simulink model "SingleTrackCANoe"  (R2021b)
settings: Solver=ode1  StartTime=0  StopTime=2  FixedStep=1.0000000000000000e-003  RelTol=1e-3
InitFcn:
  | sampleTime = str2double(get_param(bdroot, 'FixedStep'));
undefined symbols (not defined in the file or in its folder): AccPedalPos, BrakePedalPos, BrakeSwitch, DiscIntNeverNeededParam, DYNA4, EngSpd, IgnitionSwitch, InitialGear, InitialSpeed, IntendedEngTrq, LeftIndicator, MainBrakePress, MaxGear, MDL, MinGear, RefAcc, RefLane, RefLatPos, RefPath, RefPathCurv, RefSpd, RefSpdPreview, RefSpdRetrospect, RightIndicator, SteeringWheelAng, SteeringWheelTrq, UserDefinedRefValue, vm_const
libraries: UtilitiesLibrary x62, simulink x18, WheelSystemModules x14, LongitudinalControllerModules x13, LateralControllerModules x7, AnimationBusselectorModules x5, EnvironmentModules x5, BasicEngineControlModules x5, MiscellaneousControlModules x5, Animation3Modules x4, AuxiliariesModules x4, ReducedTireModules x4
(part 2 of 34)

== system SingleTrackCANoe/SimulationModel ==
  note: Update Switch Board Connections
  Enable : EnablePort  StatesWhenEnabling=reset
  Animation : Subsystem
  ComponentsOutput : Subsystem  Tag=TESIS DYNAware Interface Block  mask{NeedsUpdate=off, SignalInfo=|}
      mask SignalInfo=|
      | {
      |   "Version": "4.6",
      |   "MuxedOutputBusName": "Components",
      |   "MuxedInputBusName": "input",
      |   "MuxedInputSelected": false,
      |   "MuxedOutputSelected": true,
      |   "SignalData": [
      |     {
      |       "initialValue": "0.0",
      |       "name": "",
      |       "comment": "",
      |       "minString": "",
      |       "maxString": "",
      |       "width": 1,
      |       "dataType": 0,
      |       "signalType": 0,
      |       "createSignal": true,
      |       "outputName": "(none)",
      |       "generateSignalAccessBlock": false,
      |       "accessId": "$(parentId).$(blockName).$(outputName)"
      |     },
      |     {
      |       "initialValue": "0.0",
      |       "name": "ControlUnits",
      |       "comment": "",
      |       "minString": "",
      |       "maxString": "",
      |       "width": -1,
      |       "dataType": 0,
      |       "signalType": 1,
      |       "createSignal": false,
      |       "outputName": "ControlUnits",
      |       "generateSignalAccessBlock": false,
      |       "accessId": "$(parentId).$(blockName).$(outputName)"
      |     },
      |     {
      |       "initialValue": "0.0",
      |       "name": "Trailer",
      |       "comment": "",
      |       "minString": "",
      |       "maxString": "",
      |       "width": -1,
      |       "dataType": 0,
      |       "signalType": 1,
      |       "createSignal": false,
      |       "outputName": "Trailer",
      |       "generateSignalAccessBlock": false,
      |       "accessId": "$(parentId).$(blockName).$(outputName)"
      |     },
      |     {
      |       "initialValue": "0.0",
      |       "name": "Vehicle",
      |       "comment": "",
      |       "minString": "",
      |       "maxString": "",
      |       "width": -1,
      |       "dataType": 0,
      |       "signalType": 1,
      |       "createSignal": false,
      |       "outputName": "Vehicle",
      |       "generateSignalAccessBlock": false,
      |       "accessId": "$(parentId).$(blockName).$(outputName)"
      |     },
      |     {
      |       "initialValue": "0.0",
      |       "name": "Environment",
      |       "comment": "",
      |       "minString": "",
      |       "maxString": "",
      |       "width": -1,
      |       "dataType": 0,
      |       "signalType": 1,
      |       "createSignal": false,
      |       "outputName": "Environment",
      |       "generateSignalAccessBlock": false,
      |       "accessId": "$(parentId).$(blockName).$(outputName)"
      |     },
      |     {
      |       "initialValue": "0.0",
      |       "name": "Traffic",
      |       "comment": "",
      |       "minString": "",
      |       "maxString": "",
      |       "width": -1,
      |       "dataType": 0,
      |       "signalType": 1,
      |       "createSignal": false,
      |       "outputName": "Traffic",
      |       "generateSignalAccessBlock": false,
      |       "accessId": "$(parentId).$(blockName).$(outputName)"
      |     },
      |     {
      |       "initialValue": "0.0",
      |       "name": "VehicleControl",
      |       "comment": "",
      |       "minString": "",
      |       "maxString": "",
      |       "width": -1,
      |       "dataType": 0,
      |       "signalType": 1,
      |       "createSignal": false,
      |       "outputName": "VehicleControl",
      |       "generateSignalAccessBlock": false,
      |       "accessId": "$(parentId).$(blockName).$(outputName)"
      |     }
      |   ]
      | }
      mask prompts: NeedsUpdate "Specify, if subsystem content needs to be updated"; SignalInfo "Signal Info (json)"
      mask help: DYNA4 Interface Block Version 4.6
      mask init:
      | blockName = get_param(gcbh, 'Name');
      | parentId = DYNA4.ModelHandling.AccessID.getFromHierarchy(gcbh);
      | TD.InterfaceBlock.ModelCallbacks.GenerateContent(gcb);
      settings: AttributesFormatString=(none) = 0.0  DeleteFcn=TD.InterfaceBlock.ModelCallbacks.CloseGUI( gcbh );  NameChangeFcn=TD.InterfaceBlock.ModelCallbacks.BlockRenamedHandler(gcbh);  OpenFcn=TD.InterfaceBlock.ModelCallbacks.OpenGUI( gcbh );  CloseFcn=TD.InterfaceBlock.ModelCallbacks.CloseGUI( gcbh );
      mask Display:
      | image('InterfaceBlock.png','center');
      | port_label('input',1, 'ControlUnits');
      | port_label('input',2, 'Trailer');
      | port_label('input',3, 'Vehicle');
      | port_label('input',4, 'Environment');
      | port_label('input',5, 'Traffic');
      | port_label('input',6, 'VehicleControl');
      | port_label('output',1, 'Components');
  ControlUnits : Subsystem
  DYNA4 Logo : Subsystem
      settings: AttributesFormatString=DYNA4 Version: 9.1
      settings: PreSaveFcn=|
      | try
      |   set_param(gcb,'AttributesFormatString',['DYNA4 Version: ' dm_get_model_version(bdroot)]);
      | end
      mask Display: image('DYNA4_Model_Splash.jpg');
  Environment : Subsystem
  SwitchBoard : Subsystem  Tag=DYNA4SwitchBoard  mask{NeedsUpdate=off, SignalInfo=|}
      mask SignalInfo=|
      | {
      |   "Version": "4.6",
      |   "MuxedOutputBusName": "CTRL",
      |   "MuxedInputBusName": "Components",
      |   "MuxedInputSelected": true,
      |   "MuxedOutputSelected": true,
      |   "SignalData": [
      |     {
      |       "initialValue": "0.0",
      |       "name": "Environment.AdditionalRoadElevation.AddLatRoadSlope[-]",
      |       "comment": "",
      |       "minString": "",
      |       "maxString": "",
      |       "width": -1,
      |       "dataType": 0,
      |       "signalType": 0,
      |       "createSignal": false,
      |       "outputName": "CTRL.AdditionalRoadElevation.AddLatRoadSlope[-]",
      |       "generateSignalAccessBlock": false,
      |       "accessId": "$(outputName)"
      |     },
      |     {
      |       "initialValue": "0.0",
      |       "name": "Environment.AdditionalRoadElevation.AddLongRoadSlope[-]",
      |       "comment": "",
      |       "minString": "",
      |       "maxString": "",
      |       "width": -1,
      |       "dataType": 0,
      |       "signalType": 0,
      |       "createSignal": false,
      |       "outputName": "CTRL.AdditionalRoadElevation.AddLongRoadSlope[-]",
      |       "generateSignalAccessBlock": false,
      |       "accessId": "$(outputName)"
      |     },
      |     {
      |       "initialValue": "0.0 (auto grounded)",
      |       "name": "",
      |       "comment": "",
      |       "minString": "",
      |       "maxString": "",
      |       "width": 1,
      |       "dataType": 0,
      |       "signalType": 0,
      |       "createSignal": true,
      |       "outputName": "CTRL.AdditionalRoadElevation.ExternalAddLatRoadSlopeEnforced",
      |       "generateSignalAccessBlock": true,
      |       "accessId": "$(outputName)"
      |     },
      |     {
      |       "initialValue": "0.0 (auto grounded)",
      |       "name": "",
      |       "comment": "",
      |       "minString": "",
      |       "maxString": "",
      |       "width": 1,
      |       "dataType": 0,
      |       "signalType": 0,
      |       "createSignal": true,
      |       "outputName": "CTRL.AdditionalRoadElevation.ExternalAddLatRoadSlope[-]",
      |       "generateSignalAccessBlock": false,
      |       "accessId": "$(outputName)"
      |     },
      |     {
      |       "initialValue": "0.0 (auto grounded)",
      |       "name": "",
      |       "comment": "",
      |       "minString": "",
      |       "maxString": "",
      |       "width": 1,
      |       "dataType": 0,
      |       "signalType": 0,
      |       "createSignal": true,
      |       "outputName": "CTRL.AdditionalRoadElevation.ExternalAddLongRoadSlopeEnforced",
      |       "generateSignalAccessBlock": true,
      |       "accessId": "$(outputName)"
      |     },
      |     {
      |       "initialValue": "0.0 (auto grounded)",
      |       "name": "",
      |       "comment": "",
      |       "minString": "",
      |       "maxString": "",
      |       "width": 1,
      |       "dataType": 0,
      |       "signalType": 0,
      |       "createSignal": true,
      |       "outputName": "CTRL.AdditionalRoadElevation.ExternalAddLongRoadSlope[-]",
      |       "generateSignalAccessBlock": false,
      |       "accessId": "$(outputName)"
      |     },
      |     {
      |       "initialValue": "0.0",
      |       "name": "Environment.AdditionalRoadElevation.FrontLeftAddLatRoadSlope[-]",
      |       "comment": "",
      |       "minString": "",
      |       "maxString": "",
      |       "width": 1,
      |       "dataType": 0,
      |       "signalType": 0,
      |       "createSignal": false,
      |       "outputName": "CTRL.AdditionalRoadElevation.FrontLeftAddLatRoadSlope[-]",
      |       "generateSignalAccessBlock": false,
      |       "accessId": "$(outputName)"
      |     },
      |     {
      |       "initialValue": "0.0",
      |       "name": "Environment.AdditionalRoadElevation.FrontLeftAddLongRoadSlope[-]",
      |       "comment": "",
      |       "minString": "",
      |       "maxString": "",
      |       "width": 1,
      |       "dataType": 0,
      |       "signalType": 0,
      |       "createSignal": false,
      |       "outputName": "CTRL.AdditionalRoadElevation.FrontLeftAddLongRoadSlope[-]",
      |       "generateSignalAccessBlock": false,
      |       "accessId": "$(outputName)"
      |     },
      |     {
      |       "initialValue": "0.0",
      |       "name": "Environment.AdditionalRoadElevation.FrontLeftAddRoadElev[m]",
      |       "comment": "",
      |       "minString": "",
      |       "maxString": "",
      |       "width": -1,
      |       "dataType": 0,
      |       "signalType": 0,
      |       "createSignal": false,
      |       "outputName": "CTRL.AdditionalRoadElevation.FrontLeftAddRoadElev[m]",
      |       "generateSignalAccessBlock": false,
      |       "accessId": "$(outputName)"
      |     },
      |     {
      |       "initialValue": "0.0",
      |       "name": "Environment.AdditionalRoadElevation.FrontRightAddLatRoadSlope[-]",
      |       "comment": "",
      |       "minString": "",
      |       "maxString": "",
      |       "width": 1,
      |       "dataType": 0,
      |       "signalType": 0,
      |       "createSignal": false,
      |       "outputName": "CTRL.AdditionalRoadElevation.FrontRightAddLatRoadSlope[-]",
      |       "generateSignalAccessBlock": false,
      |       "accessId": "$(outputName)"
      |     },
      |     {
      |       "initialValue": "0.0",
      |       "name": "Environment.AdditionalRoadElevation.FrontRightAddLongRoadSlope[-]",
      |       "comment": "",
      |       "minString": "",
      |       "maxString": "",
      |       "width": 1,
      |       "dataType": 0,
      |       "signalType": 0,
      |       "createSignal": false,
      |       "outputName": "CTRL.AdditionalRoadElevation.FrontRightAddLongRoadSlope[-]",
      |       "generateSignalAccessBlock": false,
      |       "accessId": "$(outputName)"
      |     },
      |     {
      |       "initialValue": "0.0",
      |       "name": "Environment.AdditionalRoadElevation.FrontRightAddRoadElev[m]",
      |       "comment": "",
      |       "minString": "",
      |       "maxString": "",
      |       "width": -1,
      |       "dataType": 0,
      |       "signalType": 0,
      |       "createSignal": false,
      |       "outputName": "CTRL.AdditionalRoadElevation.FrontRightAddRoadElev[m]",
      |       "generateSignalAccessBlock": false,
      |       "accessId": "$(outputName)"
      |     },
      |     {
      |       "initialValue": "0.0",
      |       "name": "Environment.AdditionalRoadElevation.LocalRoadSysSwitch[0;1]",
      |       "comment": "",
      |       "minString": "",
      |       "maxString": "",
      |       "width": 1,
      |       "dataType": 0,
      |       "signalType": 0,
      |       "createSignal": false,
      |       "outputName": "CTRL.AdditionalRoadElevation.LocalRoadSysSwitch[0;1]",
      |       "generateSignalAccessBlock": false,
      |       "accessId": "$(outputName)"
      |     },
      |     {
      |       "initialValue": "0.0",
      |       "name": "Environment.AdditionalRoadElevation.RearLeftAddLatRoadSlope[-]",
      |       "comment": "",
      |       "minString": "",
      |       "maxString": "",
      |       "width": 1,
      |       "dataType": 0,
      |       "signalType": 0,
      |       "createSignal": false,
      |       "outputName": "CTRL.AdditionalRoadElevation.RearLeftAddLatRoadSlope[-]",
      |       "generateSignalAccessBlock": false,
      |       "accessId": "$(outputName)"
      |     },
      |     {
      |       "initialValue": "0.0",
      |       "name": "Environment.AdditionalRoadElevation.RearLeftAddLongRoadSlope[-]",
      |       "comment": "",
      |       "minString": "",
      |       "maxString": "",
      |       "width": 1,
      |       "dataType": 0,
      |       "signalType": 0,
      |       "createSignal": false,
      |       "outputName": "CTRL.AdditionalRoadElevation.RearLeftAddLongRoadSlope[-]",
      |       "generateSignalAccessBlock": false,
      |       "accessId": "$(outputName)"
      |     },
      |     {
      |       "initialValue": "0.0",
      |       "name": "Environment.AdditionalRoadElevation.RearLeftAddRoadElev[m]",
      |       "comment": "",
      |       "minString": "",
      |       "maxString": "",
      |       "width": 1,
      |       "dataType": 0,
      |       "signalType": 0,
      |       "createSignal": false,
      |       "outputName": "CTRL.AdditionalRoadElevation.RearLeftAddRoadElev[m]",
      |       "generateSignalAccessBlock": false,
      |       "accessId": "$(outputName)"
      |     },
      |     {
      |       "initialValue": "0.0",
      |       "name": "Environment.AdditionalRoadElevation.RearRightAddLatRoadSlope[-]",
      |       "comment": "",
      |       "minString": "",
      |       "maxString": "",
      |       "width": 1,
      |       "dataType": 0,
      |       "signalType": 0,
      |       "createSignal": false,
      |       "outputName": "CTRL.AdditionalRoadElevation.RearRightAddLatRoadSlope[-]",
      |       "generateSignalAccessBlock": false,
      |       "accessId": "$(outputName)"
      |     },
      |     {
      |       "initialValue": "0.0",
      |       "name": "Environment.AdditionalRoadElevation.RearRightAddLongRoadSlope[-]",
      |       "comment": "",
      |       "minString": "",
      |       "maxString": "",
      |       "width": 1,
      |       "dataType": 0,
      |       "signalType": 0,
      |       "createSignal": false,
      |       "outputName": "CTRL.AdditionalRoadElevation.RearRightAddLongRoadSlope[-]",
      |       "generateSignalAccessBlock": false,
      |       "accessId": "$(outputName)"
      |     },
      |     {
      |       "initialValue": "0.0",
      |       "name": "Environment.AdditionalRoadElevation.RearRightAddRoadElev[m]",
      |       "comment": "",
      |       "minString": "",
      |       "maxString": "",
      |       "width": 1,
      |       "dataType": 0,
      |       "signalType": 0,
      |       "createSignal": false,
      |       "outputName": "CTRL.AdditionalRoadElevation.RearRightAddRoadElev[m]",
      |       "generateSignalAccessBlock": false,
      |       "accessId": "$(outputName)"
      |     },
      |     {
      |       "initialValue": "0.0",
      |       "name": "Environment.AmbientConditions.AirDensity[kg/m**3]",
      |       "comment": "",
      |       "minString": "",
      |       "maxString": "",
      |       "width": 1,
      |       "dataType": 0,
      |       "signalType": 0,
      |       "createSignal": false,
      |       "outputName": "CTRL.EnvironmentalConditions.AirDensity[kg/m**3]",
      |       "generateSignalAccessBlock": false,
      |       "accessId": "$(outputName)"
      |     },
      |     {
      |       "initialValue": "0.0",
      |       "name": "Environment.AmbientConditions.AmbTemp[K]",
      |       "comment": "",
      |       "minString": "",
      |       "maxString": "",
      |       "width": 1,
      |       "dataType": 0,
      |       "signalType": 0,
      |       "createSignal": false,
      |       "outputName": "CTRL.EnvironmentalConditions.AmbTemp[K]",
      |       "generateSignalAccessBlock": false,
      |       "accessId": "$(outputName)"
      |     },
      |     {
      |       "initialValue": "0.0",
      |       "name": "Environment.RoadFrictionScaling.FrontLeftFrictionScaling[0_2]",
      |       "comment": "",
      |       "minString": "",
      |       "maxString": "",
      |       "width": 1,
      |       "dataType": 0,
      |       "signalType": 0,
      |       "createSignal": false,
      |       "outputName": "CTRL.EnvironmentalConditions.FrontLeftFrictionScaling[0_2]",
      |       "generateSignalAccessBlock": false,
      |       "accessId": "$(outputName)"
      |     },
      |     {
      |       "initialValue": "0.0",
      |       "name": "Environment.RoadFrictionScaling.FrontRightFrictionScaling[0_2]",
      |       "comment": "",
      |       "minString": "",
      |       "maxString": "",
      |       "width": 1,
      |       "dataType": 0,
      |       "signalType": 0,
      |       "createSignal": false,
      |       "outputName": "CTRL.EnvironmentalConditions.FrontRightFrictionScaling[0_2]",
      |       "generateSignalAccessBlock": false,
      |       "accessId": "$(outputName)"
      |     },
      |     {
      |       "initialValue": "0.0",
      |       "name": "Environment.RoadFrictionScaling.RearLeftFrictionScaling[0_2]",
      |       "comment": "",
      |       "minString": "",
      |       "maxString": "",
      |       "width": 1,
      |       "dataType": 0,
      |       "signalType": 0,
      |       "createSignal": false,
      |       "outputName": "CTRL.EnvironmentalConditions.RearLeftFrictionScaling[0_2]",
      |       "generateSignalAccessBlock": false,
      |       "accessId": "$(outputName)"
      |     },
      |     {
      |       "initialValue": "0.0",
      |       "name": "Environment.RoadFrictionScaling.RearRightFrictionScaling[0_2]",
      |       "comment": "",
      |       "minString": "",
      |       "maxString": "",
      |       "width": 1,
      |       "dataType": 0,
      |       "signalType": 0,
      |       "createSignal": false,
      |       "outputName": "CTRL.EnvironmentalConditions.RearRightFrictionScaling[0_2]",
      |       "generateSignalAccessBlock": false,
      |       "accessId": "$(outputName)"
      |     },
      |     {
      |       "initialValue": "0.0",
      |       "name": "Environment.WindImpact.WindDirection[rad]",
      |       "comment": "",
      |       "minString": "",
      |       "maxString": "",
      |       "width": 1,
      |       "dataType": 0,
      |       "signalType": 0,
      |       "createSignal": false,
      |       "outputName": "CTRL.EnvironmentalConditions.WindDirection[rad]",
      |       "generateSignalAccessBlock": true,
      |       "accessId": "$(outputName)"
      |     },
      |     {
      |       "initialValue": "0.0",
      |       "name": "Environment.WindImpact.WindSpd[m/s]",
      |       "comment": "",
      |       "minString": "",
      |       "maxString": "",
      |       "width": 1,
      |       "dataType": 0,
      |       "signalType": 0,
      |       "createSignal": false,
      |       "outputName": "CTRL.EnvironmentalConditions.WindSpd[m/s]",
      |       "generateSignalAccessBlock": true,
      |       "accessId": "$(outputName)"
      |     },
      |     {
      |       "initialValue": "0.0 (auto grounded)",
      |       "name": "VehicleControl.InitialConditions.InitialPitch[rad]",
      |       "comment": "",
      |       "minString": "",
      |       "maxString": "",
      |       "width": 1,
      |       "dataType": 0,
      |       "signalType": 0,
      |       "createSignal": false,
      |       "outputName": "CTRL.InitialPosition.InitialPitch[rad]",
      |       "generateSignalAccessBlock": false,
      |       "accessId": "$(outputName)"
      |     },
      |     {
      |       "initialValue": "0.0",
      |       "name": "VehicleControl.InitialConditions.InitialPositionX(WorldSys)[m]",
      |       "comment": "",
      |       "minString": "",
      |       "maxString": "",
      |       "width": 1,
      |       "dataType": 0,
      |       "signalType": 0,
      |       "createSignal": false,
      |       "outputName": "CTRL.InitialPosition.InitialPositionX(WorldSys)[m]",
      |       "generateSignalAccessBlock": false,
      |       "accessId": "$(outputName)"
      |     },
      |     {
      |       "initialValue": "0.0",
      |       "name": "VehicleControl.InitialConditions.InitialPositionY(WorldSys)[m]",
      |       "comment": "",
      |       "minString": "",
      |       "maxString": "",
      |       "width": 1,
      |       "dataType": 0,
      |       "signalType": 0,
      |       "createSignal": false,
      |       "outputName": "CTRL.InitialPosition.InitialPositionY(WorldSys)[m]",
      |       "generateSignalAccessBlock": false,
      |       "accessId": "$(outputName)"
      |     },
      |     {
      |       "initialValue": "0.0",
      |       "name": "VehicleControl.InitialConditions.InitialPositionZ(WorldSys)[m]",
      |       "comment": "",
      |       "minString": "",
      |       "maxString": "",
      |       "width": 1,
      |       "dataType": 0,
      |       "signalType": 0,
      |       "createSignal": false,
      |       "outputName": "CTRL.InitialPosition.InitialPositionZ(WorldSys)[m]",
      |       "generateSignalAccessBlock": false,
      |       "accessId": "$(outputName)"
      |     },
      |     {
      |       "initialValue": "0.0 (auto grounded)",
      |       "name": "VehicleControl.InitialConditions.InitialRoll[rad]",
      |       "comment": "",
      |       "minString": "",
      |       "maxString": "",
      |       "width": 1,
      |       "dataType": 0,
      |       "signalType": 0,
      |       "createSignal": false,
      |       "outputName": "CTRL.InitialPosition.InitialRoll[rad]",
      |       "generateSignalAccessBlock": false,
      |       "accessId": "$(outputName)"
      |     },
      |     {
      |       "initialValue": "0.0",
      |       "name": "VehicleControl.InitialConditions.InitialYaw[rad]",
      |       "comment": "",
      |       "minString": "",
      |       "maxString": "",
      |       "width": 1,
      |       "dataType": 0,
      |       "signalType": 0,
      |       "createSignal": false,
      |       "outputName": "CTRL.InitialPosition.InitialYaw[rad]",
      |       "generateSignalAccessBlock": false,
      |       "accessId": "$(outputName)"
      |     },
      |     {
      |       "initialValue": "0.0",
      |       "name": "VehicleControl.LateralControl.LateralPhase[-]",
      |       "comment": "",
      |       "minString": "",
      |       "maxString": "",
      |       "width": -1,
      |       "dataType": 0,
      |       "signalType": 0,
      |       "createSignal": false,
      |       "outputName": "CTRL.LateralControl.LateralPhase[-]",
      |       "generateSignalAccessBlock": false,
      |       "accessId": "$(outputName)"
      |     },
      |     {
      |       "initialValue": "0.0",
      |       "name": "VehicleControl.LateralControl.LeftIndicator[0;1]",
      |       "comment": "",
      |       "minString": "",
      |       "maxString": "",
      |       "width": 1,
      |       "dataType": 0,
      |       "signalType": 0,
      |       "createSignal": false,
      |       "outputName": "CTRL.LateralControl.LeftIndicator[0;1]",
      |       "generateSignalAccessBlock": true,
      |       "accessId": "$(outputName)"
      |     },
      |     {
      |       "initialValue": "0.0 (auto grounded)",
      |       "name": "",
      |       "comment": "",
      |       "minString": "",
      |       "maxString": "",
      |       "width": 1,
      |       "dataType": 0,
      |       "signalType": 0,
      |       "createSignal": true,
      |       "outputName": "CTRL.LateralControl.RefCurvEnforced",
      |       "generateSignalAccessBlock": true,
      |       "accessId": "$(outputName)"
      |     },
      |     {
      |       "initialValue": "0.0 (auto grounded)",
      |       "name": "",
      |       "comment": "",
      |       "minString": "",
      |       "maxString": "",
      |       "width": 1,
      |       "dataType": 0,
      |       "signalType": 0,
      |       "createSignal": true,
      |       "outputName": "CTRL.LateralControl.RefCurv[1/m]",
      |       "generateSignalAccessBlock": false,
      |       "accessId": "$(outputName)"
      |     },
      |     {
      |       "initialValue": "0.0 (auto grounded)",
      |       "name": "",
      |       "comment": "",
      |       "minString": "",
      |       "maxString": "",
      |       "width": 1,
      |       "dataType": 0,
      |       "signalType": 0,
      |       "createSignal": true,
      |       "outputName": "CTRL.LateralControl.RefLaneEnforced",
      |       "generateSignalAccessBlock": true,
      |       "accessId": "$(outputName)"
      |     },
      |     {
      |       "initialValue": "0.0 (auto grounded)",
      |       "name": "",
      |       "comment": "",
      |       "minString": "",
      |       "maxString": "",
      |       "width": 1,
      |       "dataType": 0,
      |       "signalType": 0,
      |       "createSignal": true,
      |       "outputName": "CTRL.LateralControl.RefLane[-]",
      |       "generateSignalAccessBlock": true,
      |       "accessId": "$(outputName)"
      |     },
      |     {
      |       "initialValue": "0.0 (auto grounded)",
      |       "name": "",
      |       "comment": "",
      |       "minString": "",
      |       "maxString": "",
      |       "width": 1,
      |       "dataType": 0,
      |       "signalType": 0,
      |       "createSignal": true,
      |       "outputName": "CTRL.LateralControl.RefLatPosEnforced",
      |       "generateSignalAccessBlock": true,
      |       "accessId": "$(outputName)"
      |     },
      |     {
      |       "initialValue": "0.0 (auto grounded)",
      |       "name": "",
      |       "comment": "",
      |       "minString": "",
      |       "maxString": "",
      |       "width": 1,
      |       "dataType": 0,
      |       "signalType": 0,
      |       "createSignal": true,
      |       "outputName": "CTRL.LateralControl.RefLatPos[m]",
      |       "generateSignalAccessBlock": false,
      |       "accessId": "$(outputName)"
      |     },
      |     {
      |       "initialValue": "0.0 (auto grounded)",
      |       "name": "",
      |       "comment": "",
      |       "minString": "",
      |       "maxString": "",
      |       "width": 1,
      |       "dataType": 0,
      |       "signalType": 0,
      |       "createSignal": true,
      |       "outputName": "CTRL.LateralControl.RefPathEnforced",
      |       "generateSignalAccessBlock": true,
      |       "accessId": "$(outputName)"
      |     },
      |     {
      |       "initialValue": "0.0 (auto grounded)",
      |       "name": "",
      |       "comment": "",
      |       "minString": "",
      |       "maxString": "",
      |       "width": 1,
      |       "dataType": 0,
      |       "signalType": 0,
      |       "createSignal": true,
      |       "outputName": "CTRL.LateralControl.RefPath[-]",
      |       "generateSignalAccessBlock": false,
      |       "accessId": "$(outputName)"
      |     },
      |     {
      |       "initialValue": "0.0",
      |       "name": "VehicleControl.LateralControl.RightIndicator[0;1]",
      |       "comment": "",
      |       "minString": "",
      |       "maxString": "",
      |       "width": 1,
      |       "dataType": 0,
      |       "signalType": 0,
      |       "createSignal": false,
      |       "outputName": "CTRL.LateralControl.RightIndicator[0;1]",
      |       "generateSignalAccessBlock": true,
      |       "accessId": "$(outputName)"
      |     },
      |     {
      |       "initialValue": "0.0",
      |       "name": "VehicleControl.LateralControl.SteeringWheelAng[rad]",
      |       "comment": "",
      |       "minString": "",
      |       "maxString": "",
      |       "width": 1,
      |       "dataType": 0,
      |       "signalType": 0,
      |       "createSignal": false,
      |       "outputName": "CTRL.LateralControl.SteeringWheelAng[rad]",
      |       "generateSignalAccessBlock": true,
      |       "accessId": "$(outputName)"
      |     },
      |     {
      |       "initialValue": "0.0",
      |       "name": "Vehicle.Chassis.FrontAxle.Steering.SteeringWheelTrq[Nm]",
      |       "comment": "",
      |       "minString": "",
      |       "maxString": "",
      |       "width": 1,
      |       "dataType": 0,
      |       "signalType": 0,
      |       "createSignal": false,
      |       "outputName": "CTRL.LateralControl.SteeringWheelTrq[Nm]",
      |       "generateSignalAccessBlock": true,
      |       "accessId": "$(outputName)"
      |     },
      |     {
      |       "initialValue": "0.0 (auto grounded)",
      |       "name": "",
      |       "comment": "",
      |       "minString": "",
      |       "maxString": "",
      |       "width": 1,
      |       "dataType": 0,
      |       "signalType": 0,
      |       "createSignal": true,
      |       "outputName": "CTRL.LateralControl.UserDefinedRefValueEnforced",
      |       "generateSignalAccessBlock": true,
      |       "accessId": "$(outputName)"
      |     },
      |     {
      |       "initialValue": "0.0 (auto grounded)",
      |       "name": "",
      |       "comment": "",
      |       "minString": "",
      |       "maxString": "",
      |       "width": 1,
      |       "dataType": 0,
      |       "signalType": 0,
      |       "createSignal": true,
      |       "outputName": "CTRL.LateralControl.UserDefinedRefValue[-]",
      |       "generateSignalAccessBlock": false,
      |       "accessId": "$(outputName)"
      |     },
      |     {
      |       "initialValue": "0.0",
      |       "name": "VehicleControl.LongitudinalControl.ABSSwitch[0;1]",
      |       "comment": "",
      |       "minString": "",
      |       "maxString": "",
      |       "width": 1,
      |       "dataType": 0,
      |       "signalType": 0,
      |       "createSignal": false,
      |       "outputName": "CTRL.LongitudinalControl.ABSSwitch[0;1]",
      |       "generateSignalAccessBlock": true,
      |       "accessId": "$(outputName)"
      |     },
      |     {
      |       "initialValue": "0.0",
      |       "name": "VehicleControl.LongitudinalControl.ACCRefSpd[m/s]",
      |       "comment": "",
      |       "minString": "",
      |       "maxString": "",
      |       "width": 1,
      |       "dataType": 0,
      |       "signalType": 0,
      |       "createSignal": false,
      |       "outputName": "CTRL.LongitudinalControl.ACCRefSpd[m/s]",
      |       "generateSignalAccessBlock": true,
      |       "accessId": "$(outputName)"
      |     },
      |     {
      |       "initialValue": "0.0",
      |       "name": "VehicleControl.LongitudinalControl.ACCSwitch[0;1]",
      |       "comment": "",
      |       "minString": "",
      |       "maxString": "",
      |       "width": 1,
      |       "dataType": 0,
      |       "signalType": 0,
      |       "createSignal": false,
      |       "outputName": "CTRL.LongitudinalControl.ACCSwitch[0;1]",
      |       "generateSignalAccessBlock": true,
      |       "accessId": "$(outputName)"
      |     },
      |     {
      |       "initialValue": "0.0",
      |       "name": "VehicleControl.LongitudinalControl.AEBSwitch[0;1]",
      |       "comment": "",
      |       "minString": "",
      |       "maxString": "",
      |       "width": 1,
      |       "dataType": 0,
      |       "signalType": 0,
      |       "createSignal": false,
      |       "outputName": "CTRL.LongitudinalControl.AEBSwitch[0;1]",
      |       "generateSignalAccessBlock": true,
      |       "accessId": "$(outputName)"
      |     },
      |     {
      |       "initialValue": "0.0",
      |       "name": "Vehicle.Drivetrain.DrivetrainControlUnit.TransmissionControlUnit.ASRRequestSwitch[0;2]",
      |       "comment": "",
      |       "minString": "",
      |       "maxString": "",
      |       "width": -1,
      |       "dataType": 0,
      |       "signalType": 0,
      |       "createSignal": false,
      |       "outputName": "CTRL.LongitudinalControl.ASRRequestSwitch[0;2]",
      |       "generateSignalAccessBlock": false,
      |       "accessId": "$(outputName)"
      |     },
      |     {
      |       "initialValue": "0.0",
      |       "name": "Vehicle.Drivetrain.DrivetrainControlUnit.TransmissionControlUnit.ASRTrq[Nm]",
      |       "comment": "",
      |       "minString": "",
      |       "maxString": "",
      |       "width": -1,
      |       "dataType": 0,
      |       "signalType": 0,
      |       "createSignal": false,
      |       "outputName": "CTRL.LongitudinalControl.ASRTrq[Nm]",
      |       "generateSignalAccessBlock": false,
      |       "accessId": "$(outputName)"
      |     },
      |     {
      |       "initialValue": "0.0",
      |       "name": "VehicleControl.LongitudinalControl.AccPedalPos[0_1]",
      |       "comment": "",
      |       "minString": "",
      |       "maxString": "",
      |       "width": 1,
      |       "dataType": 0,
      |       "signalType": 0,
      |       "createSignal": false,
      |       "outputName": "CTRL.LongitudinalControl.AccPedalPos[0_1]",
      |       "generateSignalAccessBlock": true,
      |       "accessId": "$(outputName)"
      |     },
      |     {
      |       "initialValue": "0.0",
      |       "name": "VehicleControl.LongitudinalControl.BrakePedalPos[0_1]",
      |       "comment": "",
      |       "minString": "",
      |       "maxString": "",
      |       "width": 1,
      |       "dataType": 0,
      |       "signalType": 0,
      |       "createSignal": false,
      |       "outputName": "CTRL.LongitudinalControl.BrakePedalPos[0_1]",
      |       "generateSignalAccessBlock": true,
      |       "accessId": "$(outputName)"
      |     },
      |     {
      |       "initialValue": "0.0",
      |       "name": "VehicleControl.LongitudinalControl.BrakeSwitch[1;3]",
      |       "comment": "",
      |       "minString": "",
      |       "maxString": "",
      |       "width": -1,
      |       "dataType": 0,
      |       "signalType": 0,
      |       "createSignal": false,
      |       "outputName": "CTRL.LongitudinalControl.BrakeSwitch[1;3]",
      |       "generateSignalAccessBlock": false,
      |       "accessId": "$(outputName)"
      |     },
      |     {
      |       "initialValue": "0.0",
      |       "name": "VehicleControl.LongitudinalControl.ClutchPos[0_1]",
      |       "comment": "",
      |       "minString": "",
      |       "maxString": "",
      |       "width": 1,
      |       "dataType": 0,
      |       "signalType": 0,
      |       "createSignal": false,
      |       "outputName": "CTRL.LongitudinalControl.ClutchPos[0_1]",
      |       "generateSignalAccessBlock": true,
      |       "accessId": "$(outputName)"
      |     },
      |     {
      |       "initialValue": "0.0",
      |       "name": "VehicleControl.LongitudinalControl.DayRunningLight[0;1]",
      |       "comment": "",
      |       "minString": "",
      |       "maxString": "",
      |       "width": 1,
      |       "dataType": 0,
      |       "signalType": 0,
      |       "createSignal": false,
      |       "outputName": "CTRL.LongitudinalControl.DayRunningLight[0;1]",
      |       "generateSignalAccessBlock": true,
      |       "accessId": "$(outputName)"
      |     },
      |     {
      |       "initialValue": "0.0",
      |       "name": "ControlUnits.VCU.DriverInfo.ConventionalVehicleSwitch[0;1]",
      |       "comment": "",
      |       "minString": "",
      |       "maxString": "",
      |       "width": 1,
      |       "dataType": 0,
      |       "signalType": 0,
      |       "createSignal": false,
      |       "outputName": "CTRL.LongitudinalControl.DriverInfo.ConventionalVehicleSwitch[0;1]",
      |       "generateSignalAccessBlock": false,
      |       "accessId": "$(outputName)"
      |     },
      |     {
      |       "initialValue": "0.0",
      |       "name": "Vehicle.Engine.EnginePhysics.Mechanics.MeanEngDragTrq[Nm]",
      |       "comment": "",
      |       "minString": "",
      |       "maxString": "",
      |       "width": 1,
      |       "dataType": 0,
      |       "signalType": 0,
      |       "createSignal": false,
      |       "outputName": "CTRL.LongitudinalControl.DriverInfo.MeanEngDragTrq[Nm]",
      |       "generateSignalAccessBlock": false,
      |       "accessId": "$(outputName)"
      |     },
      |     {
      |       "initialValue": "0.0",
      |       "name": "Vehicle.Engine.EnginePhysics.Mechanics.MeanEngMaxTrq[Nm]",
      |       "comment": "",
      |       "minString": "",
      |       "maxString": "",
      |       "width": 1,
      |       "dataType": 0,
      |       "signalType": 0,
      |       "createSignal": false,
      |       "outputName": "CTRL.LongitudinalControl.DriverInfo.MeanEngMaxTrq[Nm]",
      |       "generateSignalAccessBlock": false,
      |       "accessId": "$(outputName)"
      |     },
      |     {
      |       "initialValue": "0.0",
      |       "name": "Vehicle.Engine.EnginePhysics.Mechanics.ThirtyPercentAccPedalEngTrq[Nm]",
      |       "comment": "",
      |       "minString": "",
      |       "maxString": "",
      |       "width": 1,
      |       "dataType": 0,
      |       "signalType": 0,
      |       "createSignal": false,
      |       "outputName": "CTRL.LongitudinalControl.DriverInfo.ThirtyPercentAccPedalEngTrq[Nm]",
      |       "generateSignalAccessBlock": false,
      |       "accessId": "$(outputName)"
      |     },
      |     {
      |       "initialValue": "0.0 (auto grounded)",
      |       "name": "",
      |       "comment": "",
      |       "minString": "",
      |       "maxString": "",
      |       "width": 1,
      |       "dataType": 0,
      |       "signalType": 0,
      |       "createSignal": true,
      |       "outputName": "CTRL.LongitudinalControl.DriverInfo.VCUFullAccPedalTrq[Nm]",
      |       "generateSignalAccessBlock": false,
      |       "accessId": "$(outputName)"
      |     },
      |     {
      |       "initialValue": "0.0 (auto grounded)",
      |       "name": "",
      |       "comment": "",
      |       "minString": "",
      |       "maxString": "",
      |       "width": 1,
      |       "dataType": 0,
      |       "signalType": 0,
      |       "createSignal": true,
      |       "outputName": "CTRL.LongitudinalControl.DriverInfo.VCUTorqueRatio[-]",
      |       "generateSignalAccessBlock": false,
      |       "accessId": "$(outputName)"
      |     },
      |     {
      |       "initialValue": "0.0 (auto grounded)",
      |       "name": "",
      |       "comment": "",
      |       "minString": "",
      |       "maxString": "",
      |       "width": 1,
      |       "dataType": 0,
      |       "signalType": 0,
      |       "createSignal": true,
      |       "outputName": "CTRL.LongitudinalControl.DriverInfo.VCUZeroAccPedalTrq[Nm]",
      |       "generateSignalAccessBlock": false,
      |       "accessId": "$(outputName)"
      |     },
      |     {
      |       "initialValue": "0.0",
      |       "name": "VehicleControl.LongitudinalControl.ESCSwitch[0;1]",
      |       "comment": "",
      |       "minString": "",
      |       "maxString": "",
      |       "width": 1,
      |       "dataType": 0,
      |       "signalType": 0,
      |       "createSignal": false,
      |       "outputName": "CTRL.LongitudinalControl.ESCSwitch[0;1]",
      |       "generateSignalAccessBlock": true,
      |       "accessId": "$(outputName)"
      |     },
      |     {
      |       "initialValue": "0.0",
      |       "name": "ControlUnits.VCU.EngRunPermission[0;1]",
      |       "comment": "",
      |       "minString": "",
      |       "maxString": "",
      |       "width": 1,
      |       "dataType": 0,
      |       "signalType": 0,
      |       "createSignal": false,
      |       "outputName": "CTRL.LongitudinalControl.EngRunPermission[0;1]",
      |       "generateSignalAccessBlock": false,
      |       "accessId": "$(outputName)"
      |     },
      |     {
      |       "initialValue": "0.0",
      |       "name": "VehicleControl.LongitudinalControl.FogLampFront[0;1]",
      |       "comment": "",
      |       "minString": "",
      |       "maxString": "",
      |       "width": 1,
      |       "dataType": 0,
      |       "signalType": 0,
      |       "createSignal": false,
      |       "outputName": "CTRL.LongitudinalControl.FogLampFront[0;1]",
      |       "generateSignalAccessBlock": true,
      |       "accessId": "$(outputName)"
      |     },
      |     {
      |       "initialValue": "0.0",
      |       "name": "VehicleControl.LongitudinalControl.FogLampRear[0;1]",
      |       "comment": "",
      |       "minString": "",
      |       "maxString": "",
      |       "width": 1,
      |       "dataType": 0,
      |       "signalType": 0,
      |       "createSignal": false,
      |       "outputName": "CTRL.LongitudinalControl.FogLampRear[0;1]",
      |       "generateSignalAccessBlock": true,
      |       "accessId": "$(outputName)"
      |     },
      |     {
      |       "initialValue": "0.0",
      |       "name": "VehicleControl.LongitudinalControl.FrontDifferentialLock[0;1]",
      |       "comment": "",
      |       "minString": "",
      |       "maxString": "",
      |       "width": 1,
      |       "dataType": 0,
      |       "signalType": 0,
      |       "createSignal": false,
      |       "outputName": "CTRL.LongitudinalControl.FrontDifferentialLock[0;1]",
      |       "generateSignalAccessBlock": true,
      |       "accessId": "$(outputName)"
      |     },
      |     {
      |       "initialValue": "0.0",
      |       "name": "VehicleControl.LongitudinalControl.FrontLeftWheelBrakePress[Pa]",
      |       "comment": "",
      |       "minString": "",
      |       "maxString": "",
      |       "width": 1,
      |       "dataType": 0,
      |       "signalType": 0,
      |       "createSignal": false,
      |       "outputName": "CTRL.LongitudinalControl.FrontLeftWheelBrakePress[Pa]",
      |       "generateSignalAccessBlock": false,
      |       "accessId": "$(outputName)"
      |     },
      |     {
      |       "initialValue": "0.0",
      |       "name": "VehicleControl.LongitudinalControl.FrontRightWheelBrakePress[Pa]",
      |       "comment": "",
      |       "minString": "",
      |       "maxString": "",
      |       "width": 1,
      |       "dataType": 0,
      |       "signalType": 0,
      |       "createSignal": false,
      |       "outputName": "CTRL.LongitudinalControl.FrontRightWheelBrakePress[Pa]",
      |       "generateSignalAccessBlock": false,
      |       "accessId": "$(outputName)"
      |     },
      |     {
      |       "initialValue": "0.0",
      |       "name": "VehicleControl.LongitudinalControl.Handbrake[0_1]",
      |       "comment": "",
      |       "minString": "",
      |       "maxString": "",
      |       "width": 1,
      |       "dataType": 0,
      |       "signalType": 0,
      |       "createSignal": false,
      |       "outputName": "CTRL.LongitudinalControl.Handbrake[0_1]",
      |       "generateSignalAccessBlock": false,
      |       "accessId": "$(outputName)"
      |     },
      |     {
      |       "initialValue": "0.0",
      |       "name": "VehicleControl.LongitudinalControl.HighBeamLight[0;1]",
      |       "comment": "",
      |       "minString": "",
      |       "maxString": "",
      |       "width": 1,
      |       "dataType": 0,
      |       "signalType": 0,
      |       "createSignal": false,
      |       "outputName": "CTRL.LongitudinalControl.HighBeamLight[0;1]",
      |       "generateSignalAccessBlock": true,
      |       "accessId": "$(outputName)"
      |     },
      |     {
      |       "initialValue": "0.0",
      |       "name": "VehicleControl.LongitudinalControl.IgnitionSwitch[0;3]",
      |       "comment": "",
      |       "minString": "",
      |       "maxString": "",
      |       "width": 1,
      |       "dataType": 0,
      |       "signalType": 0,
      |       "createSignal": false,
      |       "outputName": "CTRL.LongitudinalControl.IgnitionSwitch[0;3]",
      |       "generateSignalAccessBlock": true,
      |       "accessId": "$(outputName)"
      |     },
      |     {
      |       "initialValue": "0.0",
      |       "name": "VehicleControl.LongitudinalControl.InitialEngineSpeed[rad/s]",
      |       "comment": "",
      |       "minString": "",
      |       "maxString": "",
      |       "width": 1,
      |       "dataType": 0,
      |       "signalType": 0,
      |       "createSignal": false,
      |       "outputName": "CTRL.LongitudinalControl.InitialEngineSpeed[rad/s]",
      |       "generateSignalAccessBlock": false,
      |       "accessId": "$(outputName)"
      |     },
      |     {
      |       "initialValue": "0.0",
      |       "name": "VehicleControl.LongitudinalControl.InitialGear[-4;20]",
      |       "comment": "",
      |       "minString": "",
      |       "maxString": "",
      |       "width": 1,
      |       "dataType": 0,
      |       "signalType": 0,
      |       "createSignal": false,
      |       "outputName": "CTRL.LongitudinalControl.InitialGear[-4;20]",
      |       "generateSignalAccessBlock": false,
      |       "accessId": "$(outputName)"
      |     },
      |     {
      |       "initialValue": "0.0",
      |       "name": "VehicleControl.LongitudinalControl.InitialSpeed[m/s]",
      |       "comment": "",
      |       "minString": "",
      |       "maxString": "",
      |       "width": 1,
      |       "dataType": 0,
      |       "signalType": 0,
      |       "createSignal": false,
      |       "outputName": "CTRL.LongitudinalControl.InitialSpeed[m/s]",
      |       "generateSignalAccessBlock": false,
      |       "accessId": "$(outputName)"
      |     },
      |     {
      |       "initialValue": "0.0",
      |       "name": "ControlUnits.VCU.IntendedEngTrqActive[0;1]",
      |       "comment": "",
      |       "minString": "",
      |       "maxString": "",
      |       "width": 1,
      |       "dataType": 0,
      |       "signalType": 0,
      |       "createSignal": false,
      |       "outputName": "CTRL.LongitudinalControl.IntendedEngTrqActive[0;1]",
      |       "generateSignalAccessBlock": false,
      |       "accessId": "$(outputName)"
      |     },
      |     {
      |       "initialValue": "0.0",
      |       "name": "VehicleControl.LongitudinalControl.IntendedEngTrq[Nm]",
      |       "comment": "",
      |       "minString": "",
      |       "maxString": "",
      |       "width": 1,
      |       "dataType": 0,
      |       "signalType": 0,
      |       "createSignal": false,
      |       "outputName": "CTRL.LongitudinalControl.IntendedEngTrq[Nm]",
      |       "generateSignalAccessBlock": false,
      |       "accessId": "$(outputName)"
      |     },
      |     {
      |       "initialValue": "0.0",
      |       "name": "VehicleControl.LongitudinalControl.KickdownSwitch[0;1]",
      |       "comment": "",
      |       "minString": "",
      |       "maxString": "",
      |       "width": 1,
      |       "dataType": 0,
      |       "signalType": 0,
      |       "createSignal": false,
      |       "outputName": "CTRL.LongitudinalControl.KickdownSwitch[0;1]",
      |       "generateSignalAccessBlock": true,
      |       "accessId": "$(outputName)"
      |     },
      |     {
      |       "initialValue": "0.0",
      |       "name": "VehicleControl.LongitudinalControl.LongitudinalPhase[-]",
      |       "comment": "",
      |       "minString": "",
      |       "maxString": "",
      |       "width": -1,
      |       "dataType": 0,
      |       "signalType": 0,
      |       "createSignal": false,
      |       "outputName": "CTRL.LongitudinalControl.LongitudinalPhase[-]",
      |       "generateSignalAccessBlock": false,
      |       "accessId": "$(outputName)"
      |     },
      |     {
      |       "initialValue": "0.0",
      |       "name": "VehicleControl.LongitudinalControl.LowBeamLight[0;1]",
      |       "comment": "",
      |       "minString": "",
      |       "maxString": "",
      |       "width": 1,
      |       "dataType": 0,
      |       "signalType": 0,
      |       "createSignal": false,
      |       "outputName": "CTRL.LongitudinalControl.LowBeamLight[0;1]",
      |       "generateSignalAccessBlock": true,
      |       "accessId": "$(outputName)"
      |     },
      |     {
      |       "initialValue": "0.0",
      |       "name": "Vehicle.Drivetrain.DrivetrainControlUnit.TransmissionControlUnit.MSRRequestSwitch[0;2]",
      |       "comment": "",
      |       "minString": "",
      |       "maxString": "",
      |       "width": -1,
      |       "dataType": 0,
      |       "signalType": 0,
      |       "createSignal": false,
      |       "outputName": "CTRL.LongitudinalControl.MSRRequestSwitch[0;2]",
      |       "generateSignalAccessBlock": false,
      |       "accessId": "$(outputName)"
      |     },
      |     {
      |       "initialValue": "0.0",
      |       "name": "Vehicle.Drivetrain.DrivetrainControlUnit.TransmissionControlUnit.MSRTrq[Nm]",
      |       "comment": "",
      |       "minString": "",
      |       "maxString": "",
      |       "width": -1,
      |       "dataType": 0,
      |       "signalType": 0,
      |       "createSignal": false,
      |       "outputName": "CTRL.LongitudinalControl.MSRTrq[Nm]",
      |       "generateSignalAccessBlock": false,
      |       "accessId": "$(outputName)"
      |     },
      |     {
      |       "initialValue": "0.0",
      |       "name": "VehicleControl.LongitudinalControl.MainBrakePress[Pa]",
      |       "comment": "",
      |       "minString": "",
      |       "maxString": "",
      |       "width": 1,
      |       "dataType": 0,
      |       "signalType": 0,
      |       "createSignal": false,
      |       "outputName": "CTRL.LongitudinalControl.MainBrakePress[Pa]",
      |       "generateSignalAccessBlock": false,
      |       "accessId": "$(outputName)"
      |     },
      |     {
      |       "initialValue": "0.0",
      |       "name": "VehicleControl.LongitudinalControl.ManualGear[-4;20]",
      |       "comment": "",
      |       "minString": "",
      |       "maxString": "",
      |       "width": 1,
      |       "dataType": 0,
      |       "signalType": 0,
      |       "createSignal": false,
      |       "outputName": "CTRL.LongitudinalControl.ManualGear[-4;20]",
      |       "generateSignalAccessBlock": true,
      |       "accessId": "$(outputName)"
      |     },
      |     {
      |       "initialValue": "0.0",
      |       "name": "VehicleControl.LongitudinalControl.AutomaticGearRange.MaxGear[-4;20]",
      |       "comment": "",
      |       "minString": "",
      |       "maxString": "",
      |       "width": 1,
      |       "dataType": 0,
      |       "signalType": 0,
      |       "createSignal": false,
      |       "outputName": "CTRL.LongitudinalControl.MaxGear[-4;20]",
      |       "generateSignalAccessBlock": true,
      |       "accessId": "$(outputName)"
      |     },
      |     {
      |       "initialValue": "0.0",
      |       "name": "VehicleControl.LongitudinalControl.AutomaticGearRange.MinGear[-4;20]",
      |       "comment": "",
      |       "minString": "",
      |       "maxString": "",
      |       "width": 1,
      |       "dataType": 0,
      |       "signalType": 0,
      |       "createSignal": false,
      |       "outputName": "CTRL.LongitudinalControl.MinGear[-4;20]",
      |       "generateSignalAccessBlock": true,
      |       "accessId": "$(outputName)"
      |     },
      |     {
      |       "initialValue": "0.0",
      |       "name": "VehicleControl.LongitudinalControl.ParkingLock[0;1]",
      |       "comment": "",
      |       "minString": "",
      |       "maxString": "",
      |       "width": 1,
      |       "dataType": 0,
      |       "signalType": 0,
      |       "createSignal": false,
      |       "outputName": "CTRL.LongitudinalControl.ParkingLock[0;1]",
      |       "generateSignalAccessBlock": false,
      |       "accessId": "$(outputName)"
      |     },
      |     {
      |       "initialValue": "0.0",
      |       "name": "VehicleControl.LongitudinalControl.Rear2DifferentialLock[0;1]",
      |       "comment": "",
      |       "minString": "",
      |       "maxString": "",
      |       "width": 1,
      |       "dataType": 0,
      |       "signalType": 0,
      |       "createSignal": false,
      |       "outputName": "CTRL.LongitudinalControl.Rear2DifferentialLock[0;1]",
      |       "generateSignalAccessBlock": false,
      |       "accessId": "$(outputName)"
      |     },
      |     {
      |       "initialValue": "0.0",
      |       "name": "VehicleControl.LongitudinalControl.Rear2LeftWheelBrakePress[Pa]",
      |       "comment": "",
      |       "minString": "",
      |       "maxString": "",
      |       "width": 1,
      |       "dataType": 0,
      |       "signalType": 0,
      |       "createSignal": false,
      |       "outputName": "CTRL.LongitudinalControl.Rear2LeftWheelBrakePress[Pa]",
      |       "generateSignalAccessBlock": false,
      |       "accessId": "$(outputName)"
      |     },
      |     {
      |       "initialValue": "0.0",
      |       "name": "VehicleControl.LongitudinalControl.Rear2RightWheelBrakePress[Pa]",
      |       "comment": "",
      |       "minString": "",
      |       "maxString": "",
      |       "width": 1,
      |       "dataType": 0,
      |       "signalType": 0,
      |       "createSignal": false,
      |       "outputName": "CTRL.LongitudinalControl.Rear2RightWheelBrakePress[Pa]",
      |       "generateSignalAccessBlock": false,
      |       "accessId": "$(outputName)"
      |     },
      |     {
      |       "initialValue": "0.0",
      |       "name": "VehicleControl.LongitudinalControl.Rear3DifferentialLock[0;1]",
      |       "comment": "",
      |       "minString": "",
      |       "maxString": "",
      |       "width": 1,
      |       "dataType": 0,
      |       "signalType": 0,
      |       "createSignal": false,
      |       "outputName": "CTRL.LongitudinalControl.Rear3DifferentialLock[0;1]",
      |       "generateSignalAccessBlock": false,
      |       "accessId": "$(outputName)"
      |     },
      |     {
      |       "initialValue": "0.0",
      |       "name": "VehicleControl.LongitudinalControl.Rear3LeftWheelBrakePress[Pa]",
      |       "comment": "",
      |       "minString": "",
      |       "maxString": "",
      |       "width": 1,
      |       "dataType": 0,
      |       "signalType": 0,
      |       "createSignal": false,
      |       "outputName": "CTRL.LongitudinalControl.Rear3LeftWheelBrakePress[Pa]",
      |       "generateSignalAccessBlock": false,
      |       "accessId": "$(outputName)"
      |     },
      |     {
      |       "initialValue": "0.0",
      |       "name": "VehicleControl.LongitudinalControl.Rear3RightWheelBrakePress[Pa]",
      |       "comment": "",
      |       "minString": "",
      |       "maxString": "",
      |       "width": 1,
      |       "dataType": 0,
      |       "signalType": 0,
      |       "createSignal": false,
      |       "outputName": "CTRL.LongitudinalControl.Rear3RightWheelBrakePress[Pa]",
      |       "generateSignalAccessBlock": false,
      |       "accessId": "$(outputName)"
      |     },
      |     {
      |       "initialValue": "0.0",
      |       "name": "VehicleControl.LongitudinalControl.RearDifferentialLock[0;1]",
      |       "comment": "",
      |       "minString": "",
      |       "maxString": "",
      |       "width": 1,
      |       "dataType": 0,
      |       "signalType": 0,
      |       "createSignal": false,
      |       "outputName": "CTRL.LongitudinalControl.RearDifferentialLock[0;1]",
      |       "generateSignalAccessBlock": true,
      |       "accessId": "$(outputName)"
      |     },
      |     {
      |       "initialValue": "0.0",
      |       "name": "VehicleControl.LongitudinalControl.RearLeftWheelBrakePress[Pa]",
      |       "comment": "",
      |       "minString": "",
      |       "maxString": "",
      |       "width": 1,
      |       "dataType": 0,
      |       "signalType": 0,
      |       "createSignal": false,
      |       "outputName": "CTRL.LongitudinalControl.RearLeftWheelBrakePress[Pa]",
      |       "generateSignalAccessBlock": false,
      |       "accessId": "$(outputName)"
      |     },
      |     {
      |       "initialValue": "0.0",
      |       "name": "VehicleControl.LongitudinalControl.RearRightWheelBrakePress[Pa]",
      |       "comment": "",
      |       "minString": "",
      |       "maxString": "",
      |       "width": 1,
      |       "dataType": 0,
      |       "signalType": 0,
      |       "createSignal": false,
      |       "outputName": "CTRL.LongitudinalControl.RearRightWheelBrakePress[Pa]",
      |       "generateSignalAccessBlock": false,
      |       "accessId": "$(outputName)"
      |     },
      |     {
      |       "initialValue": "0.0 (auto grounded)",
      |       "name": "",
      |       "comment": "",
      |       "minString": "",
      |       "maxString": "",
      |       "width": 1,
      |       "dataType": 0,
      |       "signalType": 0,
      |       "createSignal": true,
      |       "outputName": "CTRL.LongitudinalControl.RefAccEnforced",
      |       "generateSignalAccessBlock": true,
      |       "accessId": "$(outputName)"
      |     },
      |     {
      |       "initialValue": "0.0 (auto grounded)",
      |       "name": "",
      |       "comment": "",
      |       "minString": "",
      |       "maxString": "",
      |       "width": 1,
      |       "dataType": 0,
      |       "signalType": 0,
      |       "createSignal": true,
      |       "outputName": "CTRL.LongitudinalControl.RefAcc[m/s**2]",
      |       "generateSignalAccessBlock": true,
      |       "accessId": "$(outputName)"
      |     },
      |     {
      |       "initialValue": "0.0 (auto grounded)",
      |       "name": "",
      |       "comment": "",
      |       "minString": "",
      |       "maxString": "",
      |       "width": 1,
      |       "dataType": 0,
      |       "signalType": 0,
      |       "createSignal": true,
      |       "outputName": "CTRL.LongitudinalControl.RefSpdEnforced",
      |       "generateSignalAccessBlock": true,
      |       "accessId": "$(outputName)"
      |     },
      |     {
      |       "initialValue": "0.0 (auto grounded)",
      |       "name": "",
      |       "comment": "",
      |       "minString": "",
      |       "maxString": "",
      |       "width": 1,
      |       "dataType": 0,
      |       "signalType": 0,
      |       "createSignal": true,
      |       "outputName": "CTRL.LongitudinalControl.RefSpd[m/s]",
      |       "generateSignalAccessBlock": true,
      |       "accessId": "$(outputName)"
      |     },
      |     {
      |       "initialValue": "0.0",
      |       "name": "VehicleControl.LongitudinalControl.ShiftingProgramSelection[-]",
      |       "comment": "",
      |       "minString": "",
      |       "maxString": "",
      |       "width": 1,
      |       "dataType": 0,
      |       "signalType": 0,
      |       "createSignal": false,
      |       "outputName": "CTRL.LongitudinalControl.ShiftingProgramSelection[-]",
      |       "generateSignalAccessBlock": true,
      |       "accessId": "$(outputName)"
      |     },
      |     {
      |       "initialValue": "0.0",
      |       "name": "Vehicle.Engine.EngineControlUnit.StarterSwitch[0;1]",
      |       "comment": "",
      |       "minString": "",
      |       "maxString": "",
      |       "width": 1,
      |       "dataType": 0,
      |       "signalType": 0,
      |       "createSignal": false,
      |       "outputName": "CTRL.LongitudinalControl.StarterSwitch[0;1]",
      |       "generateSignalAccessBlock": false,
      |       "accessId": "$(outputName)"
      |     },
      |     {
      |       "initialValue": "0.0",
      |       "name": "VehicleControl.LongitudinalControl.TrailerFrontLeftWheelBrakePress[Pa]",
      |       "comment": "",
      |       "minString": "",
      |       "maxString": "",
      |       "width": 1,
      |       "dataType": 0,
      |       "signalType": 0,
      |       "createSignal": false,
      |       "outputName": "CTRL.LongitudinalControl.TrailerFrontLeftWheelBrakePress[Pa]",
      |       "generateSignalAccessBlock": false,
      |       "accessId": "$(outputName)"
      |     },
      |     {
      |       "initialValue": "0.0",
      |       "name": "VehicleControl.LongitudinalControl.TrailerFrontRightWheelBrakePress[Pa]",
      |       "comment": "",
      |       "minString": "",
      |       "maxString": "",
      |       "width": 1,
      |       "dataType": 0,
      |       "signalType": 0,
      |       "createSignal": false,
      |       "outputName": "CTRL.LongitudinalControl.TrailerFrontRightWheelBrakePress[Pa]",
      |       "generateSignalAccessBlock": false,
      |       "accessId": "$(outputName)"
      |     },
      |     {
      |       "initialValue": "0.0",
      |       "name": "VehicleControl.LongitudinalControl.TrailerRear2LeftWheelBrakePress[Pa]",
      |       "comment": "",
      |       "minString": "",
      |       "maxString": "",
      |       "width": 1,
      |       "dataType": 0,
      |       "signalType": 0,
      |       "createSignal": false,
      |       "outputName": "CTRL.LongitudinalControl.TrailerRear2LeftWheelBrakePress[Pa]",
      |       "generateSignalAccessBlock": false,
      |       "accessId": "$(outputName)"
      |     },
      |     {
      |       "initialValue": "0.0",
      |       "name": "VehicleControl.LongitudinalControl.TrailerRear2RightWheelBrakePress[Pa]",
      |       "comment": "",
      |       "minString": "",
      |       "maxString": "",
      |       "width": 1,
      |       "dataType": 0,
      |       "signalType": 0,
      |       "createSignal": false,
      |       "outputName": "CTRL.LongitudinalControl.TrailerRear2RightWheelBrakePress[Pa]",
      |       "generateSignalAccessBlock": false,
      |       "accessId": "$(outputName)"
      |     },
      |     {
      |       "initialValue": "0.0",
      |       "name": "VehicleControl.LongitudinalControl.TrailerRear3LeftWheelBrakePress[Pa]",
      |       "comment": "",
      |       "minString": "",
      |       "maxString": "",
      |       "width": 1,
      |       "dataType": 0,
      |       "signalType": 0,
      |       "createSignal": false,
      |       "outputName": "CTRL.LongitudinalControl.TrailerRear3LeftWheelBrakePress[Pa]",
      |       "generateSignalAccessBlock": false,
      |       "accessId": "$(outputName)"
      |     },
      |     {
      |       "initialValue": "0.0",
      |       "name": "VehicleControl.LongitudinalControl.TrailerRear3RightWheelBrakePress[Pa]",
      |       "comment": "",
      |       "minString": "",
      |       "maxString": "",
      |       "width": 1,
      |       "dataType": 0,
      |       "signalType": 0,
      |       "createSignal": false,
      |       "outputName": "CTRL.LongitudinalControl.TrailerRear3RightWheelBrakePress[Pa]",
      |       "generateSignalAccessBlock": false,
      |       "accessId": "$(outputName)"
      |     },
      |     {
      |       "initialValue": "0.0",
      |       "name": "VehicleControl.LongitudinalControl.TrailerRearLeftWheelBrakePress[Pa]",
      |       "comment": "",
      |       "minString": "",
      |       "maxString": "",
      |       "width": 1,
      |       "dataType": 0,
      |       "signalType": 0,
      |       "createSignal": false,
      |       "outputName": "CTRL.LongitudinalControl.TrailerRearLeftWheelBrakePress[Pa]",
      |       "generateSignalAccessBlock": false,
      |       "accessId": "$(outputName)"
      |     },
      |     {
      |       "initialValue": "0.0",
      |       "name": "VehicleControl.LongitudinalControl.TrailerRearRightWheelBrakePress[Pa]",
      |       "comment": "",
      |       "minString": "",
      |       "maxString": "",
      |       "width": 1,
      |       "dataType": 0,
      |       "signalType": 0,
      |       "createSignal": false,
      |       "outputName": "CTRL.LongitudinalControl.TrailerRearRightWheelBrakePress[Pa]",
      |       "generateSignalAccessBlock": false,
      |       "accessId": "$(outputName)"
      |     },
      |     {
      |       "initialValue": "0.0",
      |       "name": "VehicleControl.LongitudinalControl.TransferCaseLock[0;1]",
      |       "comment": "",
      |       "minString": "",
      |       "maxString": "",
      |       "width": 1,
      |       "dataType": 0,
      |       "signalType": 0,
      |       "createSignal": false,
      |       "outputName": "CTRL.LongitudinalControl.TransferCaseLock[0;1]",
      |       "generateSignalAccessBlock": false,
      |       "accessId": "$(outputName)"
      |     },
      |     {
      |       "initialValue": "0.0",
      |       "name": "ControlUnits.VCU.TransmissionLoad[0_1]",
      |       "comment": "",
      |       "minString": "",
      |       "maxString": "",
      |       "width": 1,
      |       "dataType": 0,
      |       "signalType": 0,
      |       "createSignal": false,
      |       "outputName": "CTRL.LongitudinalControl.TransmissionLoad[0_1]",
      |       "generateSignalAccessBlock": false,
      |       "accessId": "$(outputName)"
      |     },
      |     {
      |       "initialValue": "0.0 (auto grounded)",
      |       "name": "",
      |       "comment": "",
      |       "minString": "",
      |       "maxString": "",
      |       "width": 1,
      |       "dataType": 0,
      |       "signalType": 0,
      |       "createSignal": true,
      |       "outputName": "CTRL.LongitudinalControl.UserDefinedRefValueEnforced",
      |       "generateSignalAccessBlock": true,
      |       "accessId": "$(outputName)"
      |     },
      |     {
      |       "initialValue": "0.0 (auto grounded)",
      |       "name": "",
      |       "comment": "",
      |       "minString": "",
      |       "maxString": "",
      |       "width": 1,
      |       "dataType": 0,
      |       "signalType": 0,
      |       "createSignal": true,
      |       "outputName": "CTRL.LongitudinalControl.UserDefinedRefValue[-]",
      |       "generateSignalAccessBlock": false,
      |       "accessId": "$(outputName)"
      |     },
      |     {
      |       "initialValue": "0.0",
      |       "name": "ControlUnits.VCU.IntendedMainBrakePressActive[0;1]",
      |       "comment": "",
      |       "minString": "",
      |       "maxString": "",
      |       "width": 1,
      |       "dataType": 0,
      |       "signalType": 0,
      |       "createSignal": false,
      |       "outputName": "CTRL.LongitudinalControl.VCUIntendedMainBrakePressActive[0;1]",
      |       "generateSignalAccessBlock": false,
      |       "accessId": "$(outputName)"
      |     },
      |     {
      |       "initialValue": "0.0",
      |       "name": "ControlUnits.VCU.IntendedMainBrakePress[Pa]",
      |       "comment": "",
      |       "minString": "",
      |       "maxString": "",
      |       "width": 1,
      |       "dataType": 0,
      |       "signalType": 0,
      |       "createSignal": false,
      |       "outputName": "CTRL.LongitudinalControl.VCUIntendedMainBrakePress[Pa]",
      |       "generateSignalAccessBlock": false,
      |       "accessId": "$(outputName)"
      |     },
      |     {
      |       "initialValue": "0.0 (auto grounded)",
      |       "name": "",
      |       "comment": "",
      |       "minString": "",
      |       "maxString": "",
      |       "width": 1,
      |       "dataType": 0,
      |       "signalType": 0,
      |       "createSignal": true,
      |       "outputName": "CTRL.TireCondition.FrontLeftRelInflPress[Pa]",
      |       "generateSignalAccessBlock": false,
      |       "accessId": "$(outputName)"
      |     },
      |     {
      |       "initialValue": "0.0 (auto grounded)",
      |       "name": "",
      |       "comment": "",
      |       "minString": "",
      |       "maxString": "",
      |       "width": 1,
      |       "dataType": 0,
      |       "signalType": 0,
      |       "createSignal": true,
      |       "outputName": "CTRL.TireCondition.FrontRightRelInflPress[Pa]",
      |       "generateSignalAccessBlock": false,
      |       "accessId": "$(outputName)"
      |     },
      |     {
      |       "initialValue": "0.0 (auto grounded)",
      |       "name": "",
      |       "comment": "",
      |       "minString": "",
      |       "maxString": "",
      |       "width": 1,
      |       "dataType": 0,
      |       "signalType": 0,
      |       "createSignal": true,
      |       "outputName": "CTRL.TireCondition.RearLeftRelInflPress[Pa]",
      |       "generateSignalAccessBlock": false,
      |       "accessId": "$(outputName)"
      |     },
      |     {
      |       "initialValue": "0.0 (auto grounded)",
      |       "name": "",
      |       "comment": "",
      |       "minString": "",
      |       "maxString": "",
      |       "width": 1,
      |       "dataType": 0,
      |       "signalType": 0,
      |       "createSignal": true,
      |       "outputName": "CTRL.TireCondition.RearRightRelInflPress[Pa]",
      |       "generateSignalAccessBlock": false,
      |       "accessId": "$(outputName)"
      |     },
      |     {
      |       "initialValue": "0.0 (auto grounded)",
      |       "name": "",
      |       "comment": "",
      |       "minString": "",
      |       "maxString": "",
      |       "width": 1,
      |       "dataType": 0,
      |       "signalType": 0,
      |       "createSignal": true,
      |       "outputName": "CTRL.UserDefinedPhaseTermination.UserDefinedPhaseTermination10[-]",
      |       "generateSignalAccessBlock": false,
      |       "accessId": "$(outputName)"
      |     },
      |     {
      |       "initialValue": "0.0 (auto grounded)",
      |       "name": "",
      |       "comment": "",
      |       "minString": "",
      |       "maxString": "",
      |       "width": 1,
      |       "dataType": 0,
      |       "signalType": 0,
      |       "createSignal": true,
      |       "outputName": "CTRL.UserDefinedPhaseTermination.UserDefinedPhaseTermination1[-]",
      |       "generateSignalAccessBlock": false,
      |       "accessId": "$(outputName)"
      |     },
      |     {
      |       "initialValue": "0.0 (auto grounded)",
      |       "name": "",
      |       "comment": "",
      |       "minString": "",
      |       "maxString": "",
      |       "width": 1,
      |       "dataType": 0,
      |       "signalType": 0,
      |       "createSignal": true,
      |       "outputName": "CTRL.UserDefinedPhaseTermination.UserDefinedPhaseTermination2[-]",
      |       "generateSignalAccessBlock": false,
      |       "accessId": "$(outputName)"
      |     },
      |     {
      |       "initialValue": "0.0 (auto grounded)",
      |       "name": "",
      |       "comment": "",
      |       "minString": "",
      |       "maxString": "",
      |       "width": 1,
      |       "dataType": 0,
      |       "signalType": 0,
      |       "createSignal": true,
      |       "outputName": "CTRL.UserDefinedPhaseTermination.UserDefinedPhaseTermination3[-]",
      |       "generateSignalAccessBlock": false,
      |       "accessId": "$(outputName)"
      |     },
      |     {
      |       "initialValue": "0.0 (auto grounded)",
      |       "name": "",
      |       "comment": "",
      |       "minString": "",
      |       "maxString": "",
      |       "width": 1,
      |       "dataType": 0,
      |       "signalType": 0,
      |       "createSignal": true,
      |       "outputName": "CTRL.UserDefinedPhaseTermination.UserDefinedPhaseTermination4[-]",
      |       "generateSignalAccessBlock": false,
      |       "accessId": "$(outputName)"
      |     },
      |     {
      |       "initialValue": "0.0 (auto grounded)",
      |       "name": "",
      |       "comment": "",
      |       "minString": "",
      |       "maxString": "",
      |       "width": 1,
      |       "dataType": 0,
      |       "signalType": 0,
      |       "createSignal": true,
      |       "outputName": "CTRL.UserDefinedPhaseTermination.UserDefinedPhaseTermination5[-]",
      |       "generateSignalAccessBlock": false,
      |       "accessId": "$(outputName)"
      |     },
      |     {
      |       "initialValue": "0.0 (auto grounded)",
      |       "name": "",
      |       "comment": "",
      |       "minString": "",
      |       "maxString": "",
      |       "width": 1,
      |       "dataType": 0,
      |       "signalType": 0,
      |       "createSignal": true,
      |       "outputName": "CTRL.UserDefinedPhaseTermination.UserDefinedPhaseTermination6[-]",
      |       "generateSignalAccessBlock": false,
      |       "accessId": "$(outputName)"
      |     },
      |     {
      |       "initialValue": "0.0 (auto grounded)",
      |       "name": "",
      |       "comment": "",
      |       "minString": "",
      |       "maxString": "",
      |       "width": 1,
      |       "dataType": 0,
      |       "signalType": 0,
      |       "createSignal": true,
      |       "outputName": "CTRL.UserDefinedPhaseTermination.UserDefinedPhaseTermination7[-]",
      |       "generateSignalAccessBlock": false,
      |       "accessId": "$(outputName)"
      |     },
      |     {
      |       "initialValue": "0.0 (auto grounded)",
      |       "name": "",
      |       "comment": "",
      |       "minString": "",
      |       "maxString": "",
      |       "width": 1,
      |       "dataType": 0,
      |       "signalType": 0,
      |       "createSignal": true,
      |       "outputName": "CTRL.UserDefinedPhaseTermination.UserDefinedPhaseTermination8[-]",
      |       "generateSignalAccessBlock": false,
      |       "accessId": "$(outputName)"
      |     },
      |     {
      |       "initialValue": "0.0 (auto grounded)",
      |       "name": "",
      |       "comment": "",
      |       "minString": "",
      |       "maxString": "",
      |       "width": 1,
      |       "dataType": 0,
      |       "signalType": 0,
      |       "createSignal": true,
      |       "outputName": "CTRL.UserDefinedPhaseTermination.UserDefinedPhaseTermination9[-]",
      |       "generateSignalAccessBlock": false,
      |       "accessId": "$(outputName)"
      |     },
      |     {
      |       "initialValue": "0.0",
      |       "name": "ControlUnits.LCU.VehicleLights.BrakeLightState[0;1]",
      |       "comment": "",
      |       "minString": "",
      |       "maxString": "",
      |       "width": -1,
      |       "dataType": 0,
      |       "signalType": 0,
      |       "createSignal": false,
      |       "outputName": "CTRL.VehicleLights.BrakeLightState[0;1]",
      |       "generateSignalAccessBlock": false,
      |       "accessId": "$(outputName)"
      |     },
      |     {
      |       "initialValue": "0.0",
      |       "name": "ControlUnits.LCU.VehicleLights.DayRunningLightState[0;1]",
      |       "comment": "",
      |       "minString": "",
      |       "maxString": "",
      |       "width": -1,
      |       "dataType": 0,
      |       "signalType": 0,
      |       "createSignal": false,
      |       "outputName": "CTRL.VehicleLights.DayRunningLightState[0;1]",
      |       "generateSignalAccessBlock": false,
      |       "accessId": "$(outputName)"
      |     },
      |     {
      |       "initialValue": "0.0",
      |       "name": "ControlUnits.LCU.VehicleLights.FogLampFrontState[0;1]",
      |       "comment": "",
      |       "minString": "",
      |       "maxString": "",
      |       "width": -1,
      |       "dataType": 0,
      |       "signalType": 0,
      |       "createSignal": false,
      |       "outputName": "CTRL.VehicleLights.FogLampFrontState[0;1]",
      |       "generateSignalAccessBlock": false,
      |       "accessId": "$(outputName)"
      |     },
      |     {
      |       "initialValue": "0.0",
      |       "name": "ControlUnits.LCU.VehicleLights.FogLampRearState[0;1]",
      |       "comment": "",
      |       "minString": "",
      |       "maxString": "",
      |       "width": -1,
      |       "dataType": 0,
      |       "signalType": 0,
      |       "createSignal": false,
      |       "outputName": "CTRL.VehicleLights.FogLampRearState[0;1]",
      |       "generateSignalAccessBlock": false,
      |       "accessId": "$(outputName)"
      |     },
      |     {
      |       "initialValue": "0.0",
      |       "name": "ControlUnits.LCU.VehicleLights.HighBeamLightState[0;1]",
      |       "comment": "",
      |       "minString": "",
      |       "maxString": "",
      |       "width": -1,
      |       "dataType": 0,
      |       "signalType": 0,
      |       "createSignal": false,
      |       "outputName": "CTRL.VehicleLights.HighBeamLightState[0;1]",
      |       "generateSignalAccessBlock": false,
      |       "accessId": "$(outputName)"
      |     },
      |     {
      |       "initialValue": "0.0",
      |       "name": "ControlUnits.LCU.VehicleLights.LeftIndicatorState[0;1]",
      |       "comment": "",
      |       "minString": "",
      |       "maxString": "",
      |       "width": -1,
      |       "dataType": 0,
      |       "signalType": 0,
      |       "createSignal": false,
      |       "outputName": "CTRL.VehicleLights.LeftIndicatorState[0;1]",
      |       "generateSignalAccessBlock": false,
      |       "accessId": "$(outputName)"
      |     },
      |     {
      |       "initialValue": "0.0",
      |       "name": "ControlUnits.LCU.VehicleLights.LowBeamLightState[0;1]",
      |       "comment": "",
      |       "minString": "",
      |       "maxString": "",
      |       "width": -1,
      |       "dataType": 0,
      |       "signalType": 0,
      |       "createSignal": false,
      |       "outputName": "CTRL.VehicleLights.LowBeamLightState[0;1]",
      |       "generateSignalAccessBlock": false,
      |       "accessId": "$(outputName)"
      |     },
      |     {
      |       "initialValue": "0.0",
      |       "name": "ControlUnits.LCU.VehicleLights.ReversingLampState[0;1]",
      |       "comment": "",
      |       "minString": "",
      |       "maxString": "",
      |       "width": -1,
      |       "dataType": 0,
      |       "signalType": 0,
      |       "createSignal": false,
      |       "outputName": "CTRL.VehicleLights.ReversingLampState[0;1]",
      |       "generateSignalAccessBlock": false,
      |       "accessId": "$(outputName)"
      |     },
      |     {
      |       "initialValue": "0.0",
      |       "name": "ControlUnits.LCU.VehicleLights.RightIndicatorState[0;1]",
      |       "comment": "",
      |       "minString": "",
      |       "maxString": "",
      |       "width": -1,
      |       "dataType": 0,
      |       "signalType": 0,
      |       "createSignal": false,
      |       "outputName": "CTRL.VehicleLights.RightIndicatorState[0;1]",
      |       "generateSignalAccessBlock": false,
      |       "accessId": "$(outputName)"
      |     }
      |   ]
      | }
      mask prompts: NeedsUpdate "Specify, if subsystem content needs to be updated"; SignalInfo "Signal Info (json)"
      mask help: DYNA4 Interface Block Version 4.6
      mask init:
      | blockName = get_param(gcbh, 'Name');
      | parentId = DYNA4.ModelHandling.AccessID.getFromHierarchy(gcbh);
      | TD.InterfaceBlock.ModelCallbacks.GenerateContent(gcb);
      settings: DeleteFcn=TD.InterfaceBlock.ModelCallbacks.CloseGUI( gcbh );  NameChangeFcn=TD.InterfaceBlock.ModelCallbacks.BlockRenamedHandler(gcbh);  OpenFcn=TD.InterfaceBlock.ModelCallbacks.OpenGUI( gcbh );  CloseFcn=TD.InterfaceBlock.ModelCallbacks.CloseGUI( gcbh );
      mask Display: image('SwitchBoard.png','center');
  TraceMarker : UtilitiesLibrary/DYNA4 Trace Marker  Tag=DYNA4_TRACE_MARKER  SettingType=Standard  PrefixModelBlockID=on  PrefixRootSignalName=off  NamePattern='$(modelBlockID).$(rootSignalName)'
  Traffic : Subsystem
  Trailer : Subsystem
  Vehicle : Subsystem
  VehicleControl : Subsystem  LoadFcn=|
      | DYNA4.VehicleControl.BusObjects.Create_TD_BO_LongitudinalControlInputs
      | DYNA4.VehicleControl.BusObjects.Create_TD_BO_LateralControlInputs
      | DYNA4.VehicleControl.BusObjects.Create_TD_BO_LongitudinalSpeedControlOutputs
  wires:
  Traffic/1(Traffic) -> ComponentsOutput/5(Traffic___UNIQUE_1), VehicleControl/4(fromTraffic), ControlUnits/4(fromTraffic), Animation/5(fromTraffic), Environment/4(fromTraffic)  "Traffic"
  ComponentsOutput/1(Components___UNIQUE_1) -> SwitchBoard/1(Components)
  Vehicle/1(Vehicle) -> ComponentsOutput/3(Vehicle___UNIQUE_1), ControlUnits/3(fromVehicle), Animation/4(fromVehicle), Trailer/2(fromVehicle), VehicleControl/3(fromVehicle), Traffic/2(fromVehicle), Environment/3(fromVehicle)  "Vehicle"
  ControlUnits/1(ControlUnits) -> ComponentsOutput/1(ControlUnits___UNIQUE_1), Animation/2(fromControlUnits)  "ControlUnits"
  SwitchBoard/1(CTRL___UNIQUE_1) -> VehicleControl/1(fromCTRL), ControlUnits/1(fromCTRL), Animation/1(fromCTRL), Trailer/1(fromCTRL), Vehicle/1(fromCTRL), Environment/1(fromCTRL), Traffic/1(fromCTRL), TraceMarker/1
  VehicleControl/1(VehicleControl) -> ComponentsOutput/6(VehicleControl___UNIQUE_1)  "VehicleControl"
  Environment/1(Environment) -> ComponentsOutput/4(Environment___UNIQUE_1), Vehicle/3(fromEnvironment)  "Environment"
  Trailer/1(Trailer) -> ComponentsOutput/2(Trailer___UNIQUE_1), Vehicle/2(fromTrailer), VehicleControl/2(fromTrailer), Environment/2(fromTrailer), ControlUnits/2(fromTrailer), Animation/3(fromTrailer)  "Trailer"
